simulink model "SS_tracking2"  (R2024b)
settings: Solver=ode1  StartTime=0.0  StopTime=inf  FixedStep=0.002  RelTol=1e-3  EnableMultiTasking=on
PostLoadFcn:
  | qc_set_target_type(getConfigSet(bdroot, 'QUARC Default Target Configuration'));
undefined symbols (not defined in the file): A_sw, Aobs, Aobs_d, B_sw, Bobs, Bobs_d, C_sw, Cobs, Cobs_d, D_sw, Dobs, HIL, init_cond4, K4, theta_ref_amp, theta_ref_bias, theta_ref_freq, theta_ref_phase, thetaddot_ref_amp, thetaddot_ref_bias, thetaddot_ref_freq, thetaddot_ref_phase, thetadot_ref_amp, thetadot_ref_bias, thetadot_ref_freq, thetadot_ref_phase, ud_neg, ud_pos, uff_theta_gain, uff_thetaddot_gain, uff_thetadot_gain, uff_xc_gain, uff_xcdot_gain, V_sat, xc_ref_amp, xc_ref_bias, xc_ref_freq, xc_ref_phase, xcdot_ref_amp, xcdot_ref_bias, xcdot_ref_freq, xcdot_ref_phase
libraries: quarc_library x4, cstblocks x4, simulink_extras x1
settings Model: SimulationMode=external  ExtModeTrigDuration=5000  Creator=pmartin  LastModifiedBy=Student
settings SolverCC: AlgebraicLoopSolver=TrustRegion  PositivePriorityOrder=on
settings DataIOCC: LimitDataPoints=on  SaveFormat=Array  SignalLoggingSaveFormat=ModelDataLogs  ReturnWorkspaceOutputs=off
settings OptimizationCC: ExpressionDepthLimit=2147483647  InitFltsAndDblsToZero=on
settings DebuggingCC: SaveWithParameterizedLinksMsg=none  UnderspecifiedInitializationDetection=Classic  MergeDetectMultiDrivingBlocksExec=none  SolverPrmCheckMsg=warning  MultiTaskDSMMsg=warning  MultiTaskCondExecSysMsg=none  FcnCallInpInsideContextMsg=warning  UnconnectedInputMsg=warning  UnconnectedOutputMsg=warning  UnconnectedLineMsg=warning  StateNameClashWarn=warning  SFUnexpectedBacktrackingDiag=warning  SFNoUnconditionalDefaultTransitionDiag=warning  SFExecutionAtInitializationDiag=none  ArithmeticOperatorsInVariantConditions=warning
settings ModelReferenceCC: PropagateSignalLabelsOutOfModel=off
settings SFSimCC: SimUseLocalCustomCode=off  CustomCodeUndefinedFunction=UseInterfaceOnly
settings RTWCC: Description=QUARC Win64 Target Using Toolchain  SystemTargetFile=quarc_win64.tlc  TemplateMakefile=quarc_default_tmf  RTWUseLocalCustomCode=off  Toolchain=QUARC win64 | nmake (64-bit Windows)  BuildConfiguration=Faster Runs  GPUComputeCapability=3.5
settings CodeAppCC: StateflowObjectComments=on
settings STFCustomTargetCC: ConcurrentExecutionCompliant=on  GRTInterface=on  UseToolchainInfoCompliant=on  SystemTargetFile=quarc_win64.tlc
settings GRTTargetCC: TargetLangStandard=C89/C90 (ANSI)  ParMdlRefBuildCompliant=off  CompOptLevelCompliant=off  CombineOutputUpdateFcns=off  MatFileLogging=off  CPPClassGenCompliant=off  GRTInterface=on  ExtMode=on  ExtModeMexFile=quarc_comm
settings ConfigComp: CovMetricSettings=dw  CovSaveCumulativeToWorkspaceVar=on  CovSaveSingleToWorkspaceVar=on  CovExternalEMLEnable=off

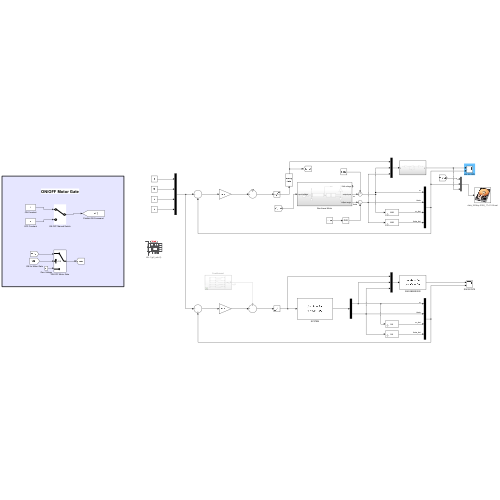
[thumbnail: Simulink's stored preview of the top-level diagram]
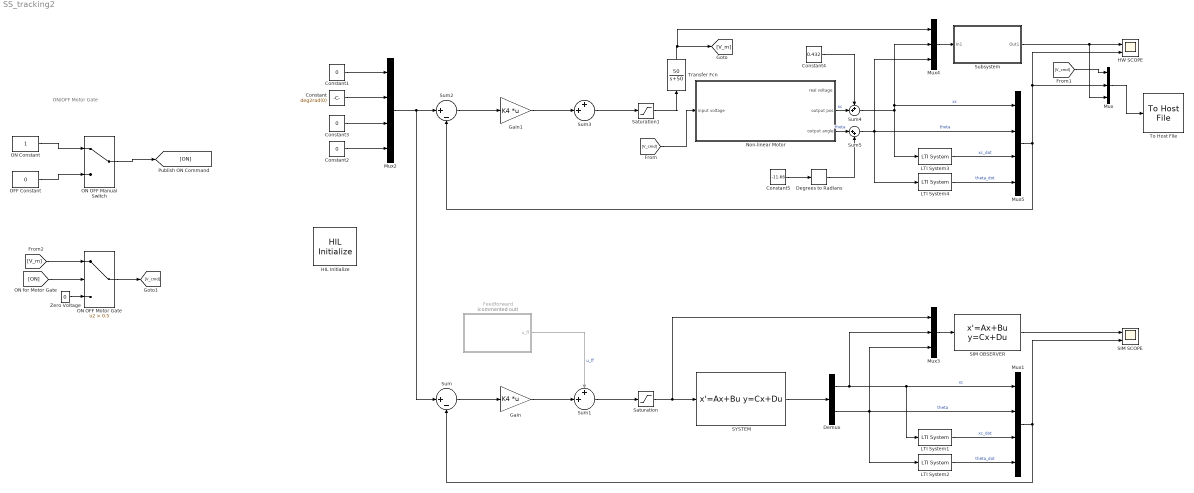
== system SS_tracking2 ==
  note: ON/OFF Motor Gate
  Constant : Constant  Value=deg2rad(0)
  Constant1 : Constant  Value=0
  Constant2 : Constant  Value=0
  Constant3 : Constant  Value=0
  Constant4 : Constant  Value=0.432
  Constant5 : Constant  Value=-11.66
  Degrees to Radians : simulink_extras/Transformations/Degrees to Radians
  Demux : Demux  Outputs=2
  Feedforward : Subsystem  Commented=on
  Gain : Gain  Gain=K4  Multiplication=Matrix(K*u)
  Gain1 : Gain  Gain=K4  Multiplication=Matrix(K*u)
  HIL Initialize : quarc_library/Data Acquisition/Generic/Configuration/HIL Initialize  object_name=HIL-1  board_type=q2_usb  board_number=0  board_options=d0=digital;d1=digital;led=auto;update_rate=normal  exclusive=off  active=off  hardware_clocks=[0:2]  clock_modes=[]  initial_clock_frequencies=[]  set_clock_params_at_start=off  set_clock_params_at_switch_in=off  set_clock_frequencies_at_start=off  set_clock_frequencies_at_switch_in=off  analog_input_channels=[0:1]  analog_input_configurations=[]  analog_input_maximums=10  analog_input_minimums=-10  set_analog_input_params_at_start=on  set_analog_input_params_at_switch_in=off  analog_output_channels=[0:1]  analog_output_maximums=10  analog_output_minimums=-10  initial_analog_outputs=[0]  final_analog_outputs=[0]  watchdog_analog_outputs=0  set_analog_output_params_at_start=on  set_analog_output_params_at_switch_in=off  set_analog_outputs_at_start=on  set_analog_outputs_at_switch_in=off  set_analog_outputs_at_terminate=on  set_analog_outputs_at_switch_out=off  set_analog_outputs_on_watchdog=off  digital_input_channels=[]  digital_output_channels=[0:7]  digital_output_configuration=[]  initial_digital_outputs=[0]  final_digital_outputs=[0]  watchdog_digital_outputs=[0]  set_digital_output_params_at_start=off  set_digital_output_params_at_switch_in=off  set_digital_outputs_at_start=on  set_digital_outputs_at_switch_in=off  set_digital_outputs_at_terminate=on  set_digital_outputs_at_switch_out=off  set_digital_outputs_on_watchdog=off  encoder_channels=[0:1]  quadrature=[4]  encoder_filter_frequency=[]  initial_encoder_counts=[0]  set_encoder_params_at_start=on  set_encoder_params_at_switch_in=off  set_encoder_counts_at_start=on  set_encoder_counts_at_switch_in=off  pwm_channels=[]  pwm_modes=[0]  pwm_frequency=1/0.020  pwm_configuration=[]  pwm_alignment=[]  pwm_polarity=[]  pwm_leading_deadband=[]  pwm_trailing_deadband=[]  initial_pwm_outputs=[0]  final_pwm_outputs=[0]  watchdog_pwm_outputs=[0]  set_pwm_params_at_start=on  set_pwm_params_at_switch_in=off  set_pwm_outputs_at_start=on  set_pwm_outputs_at_switch_in=off  set_pwm_outputs_at_terminate=on  set_pwm_outputs_at_switch_out=off  set_pwm_outputs_on_watchdog=off  other_output_channels=[]  initial_other_outputs=[]  final_other_outputs=[]  watchdog_other_outputs=[]  set_other_outputs_at_start=off  set_other_outputs_at_switch_in=off  set_other_outputs_at_terminate=off  set_other_outputs_at_switch_out=off  set_other_outputs_on_watchdog=off
  HW SCOPE : Scope  NumInputPorts=2
  LTI System1 : cstblocks/LTI System  sys=H4  IC=[]  PadeOrder=0
  LTI System2 : cstblocks/LTI System  sys=H4  IC=[]  PadeOrder=0
  LTI System3 : cstblocks/LTI System  sys=H4d  IC=[]  PadeOrder=0
  LTI System4 : cstblocks/LTI System  sys=H4d  IC=[]  PadeOrder=0
  Mux : Mux  Inputs=3
  Mux1 : Mux
  Mux2 : Mux
  Mux3 : Mux  Inputs=3
  Mux4 : Mux  Inputs=3
  Mux5 : Mux
  Non-linear Motor : Subsystem
  OFF Constant : Constant  Value=0
  ON Constant : Constant
  ON OFF Manual Switch : ManualSwitch
  ON OFF Motor Gate : Switch  Criteria=u2 > Threshold  Threshold=0.5  SaturateOnIntegerOverflow=off  InputSameDT=off
  SIM OBSERVER : StateSpace  A=Aobs  B=Bobs  C=Cobs  D=Dobs  InitialCondition=init_cond4
  SIM SCOPE : Scope  NumInputPorts=2
  SYSTEM : StateSpace  A=A_sw  B=B_sw  C=C_sw  D=D_sw  InitialCondition=init_cond4
  Saturation : Saturate  UpperLimit=V_sat - ud_pos  LowerLimit=-V_sat + ud_neg
  Saturation1 : Saturate  UpperLimit=V_sat - ud_pos  LowerLimit=-V_sat + ud_neg
  Subsystem : Subsystem
  Sum : Sum  Inputs=|+-
  Sum1 : Sum  Inputs=++|
  Sum2 : Sum  Inputs=|+-
  Sum3 : Sum  Inputs=++|
  Sum4 : Sum  Inputs=++|
  Sum5 : Sum  Inputs=|++
  To Host File : quarc_library/Sinks/To Host/To Host File  source=Specify via dialog (do not evaluate)  file_name=data_%{date}_%{time}.mat  variable_name=data  decimation=1  sample_time=-1  file_format=MAT-file v.4  options=No header or footer  append=off  final_file_name=data_26-May-2026_17-41-59.mat  encoding=Default  bitrate=0
  Transfer Fcn : TransferFcn  Numerator=50  Denominator=[1 50]
  Zero Voltage : Constant  Value=0
  wires:
  SYSTEM/1 -> Demux/1
  Demux/1 -> Mux3/2, LTI System1/1, Mux1/1  "xc"
  Demux/2 -> Mux3/3, LTI System2/1, Mux1/2  "theta"
  LTI System1/1 -> Mux1/3  "xc_dot"
  LTI System2/1 -> Mux1/4  "theta_dot"
  Saturation/1 -> Mux3/1, SYSTEM/1
  Sum/1 -> Gain/1
  Mux1/1 -> Sum/2, SIM SCOPE/2
  Mux2/1 -> Sum2/1, Sum/1
  Sum1/1 -> Saturation/1
  Gain/1 -> Sum1/2
  Constant1/1 -> Mux2/1
  Constant/1 -> Mux2/2
  Constant3/1 -> Mux2/3
  Constant2/1 -> Mux2/4
  Mux3/1 -> SIM OBSERVER/1
  SIM OBSERVER/1 -> SIM SCOPE/1
  Feedforward/1(u_ff) -> Sum1/1  "u_ff"
  Gain1/1 -> Sum3/2
  Sum3/1 -> Saturation1/1
  Sum2/1 -> Gain1/1
  Mux4/1 -> Subsystem/1(In1)
  Sum4/1 -> Mux4/2, Mux5/1, LTI System3/1  "xc"
  Sum5/1 -> LTI System4/1, Mux4/3, Mux5/2  "theta"
  LTI System3/1 -> Mux5/3  "xc_dot"
  LTI System4/1 -> Mux5/4  "theta_dot"
  Saturation1/1 -> Transfer Fcn/1
  Subsystem/1(Out1) -> Mux/3, HW SCOPE/1
  Mux5/1 -> HW SCOPE/2, Mux/2, Sum2/2
  Mux/1 -> To Host File/1
  [V_m] -> ON OFF Motor Gate/1
  [ON] -> ON OFF Motor Gate/2
  Zero Voltage/1 -> ON OFF Motor Gate/3
  ON OFF Motor Gate/1 -> [V_cmd]
  OFF Constant/1 -> ON OFF Manual Switch/2
  ON Constant/1 -> ON OFF Manual Switch/1
  ON OFF Manual Switch/1 -> [ON]
  [V_cmd] -> Non-linear Motor/1(input voltage)
  [V_cmd] -> Mux/1
  Non-linear Motor/2(output pos) -> Sum4/2  "xc"
  Constant4/1 -> Sum4/1
  Constant5/1 -> Degrees to Radians/1
  Non-linear Motor/3(output angle) -> Sum5/1  "theta"
  Degrees to Radians/1 -> Sum5/2
  Transfer Fcn/1 -> [V_m], Mux4/1

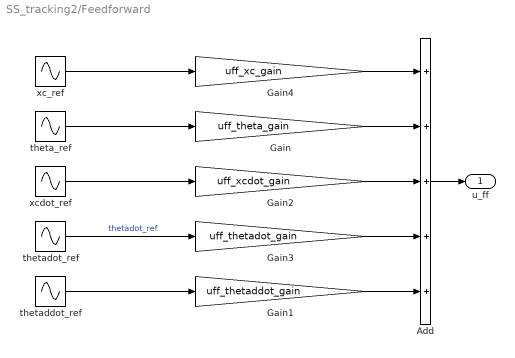
== system SS_tracking2/Feedforward ==
  Add : Sum  Inputs=+++++
  Gain : Gain  Gain=uff_theta_gain
  Gain1 : Gain  Gain=uff_thetaddot_gain
  Gain2 : Gain  Gain=uff_xcdot_gain
  Gain3 : Gain  Gain=uff_thetadot_gain
  Gain4 : Gain  Gain=uff_xc_gain
  theta_ref : Sin  Amplitude=theta_ref_amp  Bias=theta_ref_bias  Frequency=theta_ref_freq  Phase=theta_ref_phase  SampleTime=0
  thetaddot_ref : Sin  Amplitude=thetaddot_ref_amp  Bias=thetaddot_ref_bias  Frequency=thetaddot_ref_freq  Phase=thetaddot_ref_phase  SampleTime=0
  thetadot_ref : Sin  Amplitude=thetadot_ref_amp  Bias=thetadot_ref_bias  Frequency=thetadot_ref_freq  Phase=thetadot_ref_phase  SampleTime=0
  xc_ref : Sin  Amplitude=xc_ref_amp  Bias=xc_ref_bias  Frequency=xc_ref_freq  Phase=xc_ref_phase  SampleTime=0
  xcdot_ref : Sin  Amplitude=xcdot_ref_amp  Bias=xcdot_ref_bias  Frequency=xcdot_ref_freq  Phase=xcdot_ref_phase  SampleTime=0
  u_ff : Outport
  wires:
  theta_ref/1 -> Gain/1
  Gain/1 -> Add/2
  thetaddot_ref/1 -> Gain1/1
  Gain1/1 -> Add/5
  Add/1 -> u_ff/1
  Gain2/1 -> Add/3
  xcdot_ref/1 -> Gain2/1
  Gain3/1 -> Add/4
  Gain4/1 -> Add/1
  xc_ref/1 -> Gain4/1
  thetadot_ref/1 -> Gain3/1  "thetadot_ref"

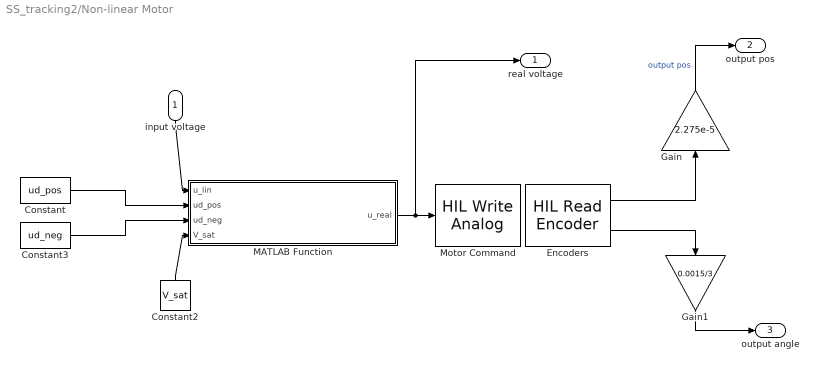
== system SS_tracking2/Non-linear Motor ==
  input voltage : Inport
  Constant : Constant  Value=ud_pos
  Constant2 : Constant  Value=V_sat
  Constant3 : Constant  Value=ud_neg
  Encoders : quarc_library/Data Acquisition/Generic/Immediate I//O/HIL Read Encoder  object_name=HIL-1  channels=[0,1]  sample_time=qc_get_step_size  active=on  vector_output=off  data_type_mode=Inherit via back propagation  data_type=double
  Gain : Gain  Gain=2.275e-5
  Gain1 : Gain  Gain=0.0015/3
  MATLAB Function : MATLAB Function  TreatAsAtomicUnit=on
  Motor Command : quarc_library/Data Acquisition/Generic/Immediate I//O/HIL Write Analog  object_name=HIL-1  channels=0  sample_time=-1  active=off  vector_input=off
  real voltage : Outport
  output pos : Outport  Port=2
  output angle : Outport  Port=3
  wires:
  Encoders/1 -> Gain/1
  input voltage/1 -> MATLAB Function/1(u_lin)
  Gain/1 -> output pos/1  "output pos"
  MATLAB Function/1(u_real) -> real voltage/1, Motor Command/1
  Constant/1 -> MATLAB Function/2(ud_pos)
  Constant3/1 -> MATLAB Function/3(ud_neg)
  Constant2/1 -> MATLAB Function/4(V_sat)
  Encoders/2 -> Gain1/1
  Gain1/1 -> output angle/1

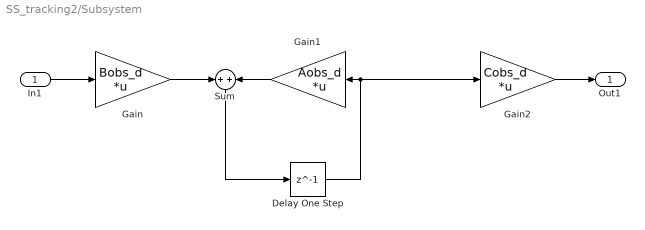
== system SS_tracking2/Subsystem ==
  In1 : Inport
  Delay One Step : Delay  DelayLength=1
  Gain : Gain  Gain=Bobs_d  Multiplication=Matrix(K*u)
  Gain1 : Gain  Gain=Aobs_d  Multiplication=Matrix(K*u)
  Gain2 : Gain  Gain=Cobs_d  Multiplication=Matrix(K*u)
  Sum : Sum  Inputs=+|+
  Out1 : Outport
  wires:
  In1/1 -> Gain/1
  Gain/1 -> Sum/1
  Gain2/1 -> Out1/1
  Sum/1 -> Delay One Step/1
  Gain1/1 -> Sum/2
  Delay One Step/1 -> Gain2/1, Gain1/1

== matlab function SS_tracking2/Non-linear Motor/MATLAB Function ==
  data: u_lin input; u_real output; ud_pos input; ud_neg input; V_sat input
function u_real = non_linear_deadzone(u_lin, ud_pos, ud_neg, V_sat)

epsilon = 0.1;

if u_lin > epsilon
    u_real = u_lin + ud_pos;
    
elseif u_lin < -epsilon
    u_real = u_lin - ud_neg;
    
else
    u_real = 0;
end

if u_real > V_sat
    u_real = V_sat;
elseif u_real < -V_sat
    u_real = -V_sat;
end
